simulink model "Control_System_Integrated"  (R2024a)
settings: Solver=ode23tb  StartTime=0.0  StopTime=0.1  FixedStep=1e-5  MaxStep=1e-05  RelTol=1e-3
settings Model: Creator=PME406_01  LastModifiedBy=PME406_01

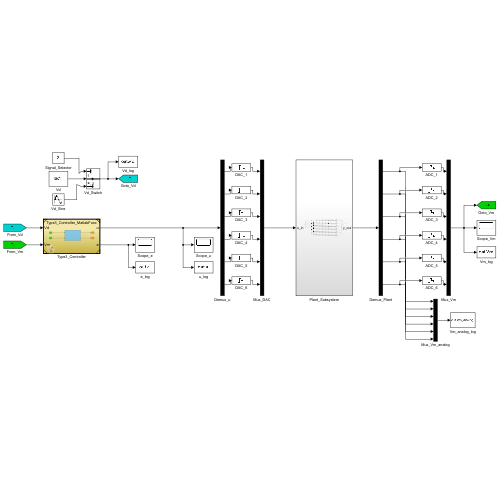
[thumbnail: Simulink's stored preview of the top-level diagram]
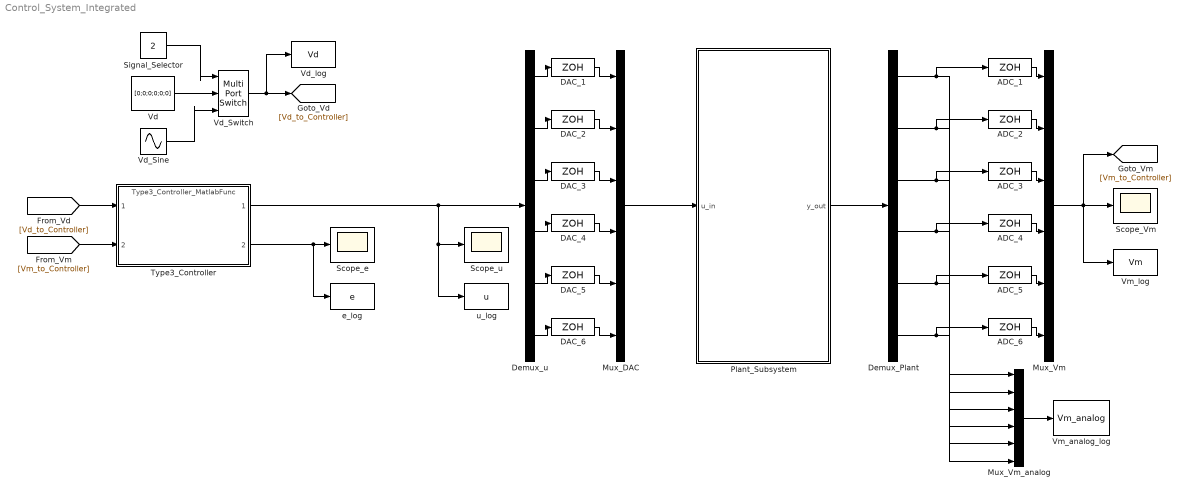
== system Control_System_Integrated ==
  ADC_{1..6} (6 alike) : ZeroOrderHold  SampleTime=1e-05
  DAC_{1..6} (6 alike) : ZeroOrderHold  SampleTime=1e-05
  Demux_Plant : Demux  Outputs=6
  Demux_u : Demux  Outputs=6
  Mux_DAC : Mux  Inputs=6
  Mux_Vm : Mux  Inputs=6
  Mux_Vm_analog : Mux  Inputs=6
  Plant_Subsystem : Subsystem
  Scope_Vm : Scope
  Scope_e : Scope
  Scope_u : Scope
  Signal_Selector : Constant  Value=2
  Type3_Controller : ModelReference  ModelNameDialog=Type3_Controller_MatlabFunc  SimulationMode=Normal  ModelReferenceVersion=1.12
  Vd : Constant  Value=[0;0;0;0;0;0]  SampleTime=1e-05
  Vd_Sine : Sin  Amplitude=[0;0;0;0;0.5;0]  Bias=[0; 0; 0; 0; 0; 0]  Frequency=3141.5927  Phase=[0;0;0;0;0;0]  SampleTime=1e-5
  Vd_Switch : MultiPortSwitch  Inputs=2  SaturateOnIntegerOverflow=off  InputSameDT=off
  Vd_log : ToWorkspace  VariableName=Vd  SampleTime=-1
      settings: Save2DSignal=2-D array (concatenate along first dimension)
  Vm_analog_log : ToWorkspace  VariableName=Vm_analog  SampleTime=-1
      settings: Save2DSignal=2-D array (concatenate along first dimension)
  Vm_log : ToWorkspace  VariableName=Vm  SampleTime=-1
      settings: Save2DSignal=2-D array (concatenate along first dimension)
  e_log : ToWorkspace  VariableName=e  SampleTime=-1
      settings: Save2DSignal=2-D array (concatenate along first dimension)
  u_log : ToWorkspace  VariableName=u  SampleTime=-1
      settings: Save2DSignal=2-D array (concatenate along first dimension)
  wires:
  Type3_Controller/1 -> u_log/1, Scope_u/1, Demux_u/1
  Demux_u/1 -> DAC_1/1
  Demux_u/2 -> DAC_2/1
  Demux_u/3 -> DAC_3/1
  Demux_u/4 -> DAC_4/1
  Demux_u/5 -> DAC_5/1
  Demux_u/6 -> DAC_6/1
  DAC_1/1 -> Mux_DAC/1
  DAC_2/1 -> Mux_DAC/2
  DAC_3/1 -> Mux_DAC/3
  DAC_4/1 -> Mux_DAC/4
  DAC_5/1 -> Mux_DAC/5
  DAC_6/1 -> Mux_DAC/6
  Plant_Subsystem/1(y_out) -> Demux_Plant/1
  Demux_Plant/1 -> ADC_1/1, Mux_Vm_analog/1
  Demux_Plant/2 -> ADC_2/1, Mux_Vm_analog/2
  Demux_Plant/3 -> ADC_3/1, Mux_Vm_analog/3
  Demux_Plant/4 -> ADC_4/1, Mux_Vm_analog/4
  Demux_Plant/5 -> ADC_5/1, Mux_Vm_analog/5
  Demux_Plant/6 -> ADC_6/1, Mux_Vm_analog/6
  ADC_1/1 -> Mux_Vm/1
  ADC_2/1 -> Mux_Vm/2
  ADC_3/1 -> Mux_Vm/3
  ADC_4/1 -> Mux_Vm/4
  ADC_5/1 -> Mux_Vm/5
  ADC_6/1 -> Mux_Vm/6
  Mux_Vm/1 -> Vm_log/1, Scope_Vm/1, [Vm_to_Controller]
  Mux_Vm_analog/1 -> Vm_analog_log/1
  Type3_Controller/2 -> e_log/1, Scope_e/1
  [Vm_to_Controller] -> Type3_Controller/2
  [Vd_to_Controller] -> Type3_Controller/1
  Vd/1 -> Vd_Switch/2
  Vd_Sine/1 -> Vd_Switch/3
  Signal_Selector/1 -> Vd_Switch/1
  Vd_Switch/1 -> Vd_log/1, [Vd_to_Controller]
  Mux_DAC/1 -> Plant_Subsystem/1(u_in)

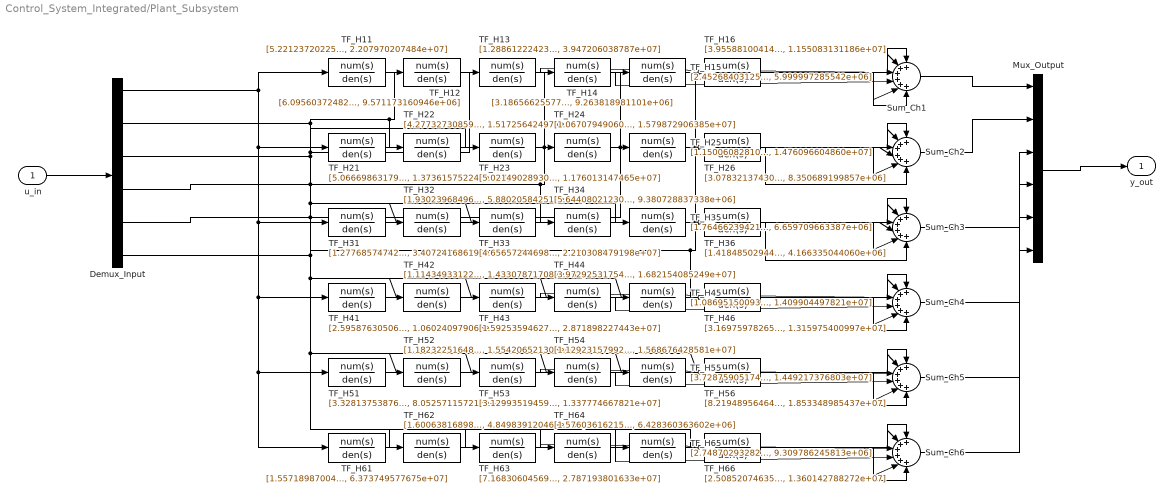
== system Control_System_Integrated/Plant_Subsystem ==
  u_in : Inport
  Demux_Input : Demux  Outputs=6
  Mux_Output : Mux  Inputs=6
  Sum_Ch{1..6} (6 alike) : Sum  Inputs=++++++
  TF_H11 : TransferFcn  Numerator=[5.221237202258e+06]  Denominator=[1, 1.125476429798e+04, 2.207970207484e+07]
  TF_H12 : TransferFcn  Numerator=[6.095603724823e+04]  Denominator=[1, 1.615096196557e+03, 9.571173160946e+06]
  TF_H13 : TransferFcn  Numerator=[1.288612224236e+06]  Denominator=[1, 1.231137597589e+04, 3.947206038787e+07]
  TF_H14 : TransferFcn  Numerator=[3.186566255776e+05]  Denominator=[1, 7.765927137710e+03, 9.263818981101e+06]
  TF_H15 : TransferFcn  Numerator=[2.452684031253e+05]  Denominator=[1, 5.746401647961e+03, 5.999997285542e+06]
  TF_H16 : TransferFcn  Numerator=[3.955881004140e+05]  Denominator=[1, 3.580306515557e+03, 1.155083131186e+07]
  TF_H21 : TransferFcn  Numerator=[5.066698631790e+04]  Denominator=[1, 1.108261849372e+03, 1.373615752245e+07]
  TF_H22 : TransferFcn  Numerator=[4.277327308593e+06]  Denominator=[1, 1.003268373777e+04, 1.517256424974e+07]
  TF_H23 : TransferFcn  Numerator=[5.021490289304e+05]  Denominator=[1, 8.810895080316e+03, 1.176013147465e+07]
  TF_H24 : TransferFcn  Numerator=[1.067079490600e+06]  Denominator=[1, 1.135112820448e+04, 1.579872906385e+07]
  TF_H25 : TransferFcn  Numerator=[1.150060828107e+06]  Denominator=[1, 1.065992916636e+04, 1.476096604860e+07]
  TF_H26 : TransferFcn  Numerator=[3.078321374306e+05]  Denominator=[1, 6.847783968129e+03, 8.350689199857e+06]
  TF_H31 : TransferFcn  Numerator=[1.277685747428e+06]  Denominator=[1, 1.368269686933e+04, 3.407241686199e+07]
  TF_H32 : TransferFcn  Numerator=[1.930239684968e+05]  Denominator=[1, 4.560870597302e+03, 5.880205842512e+06]
  TF_H33 : TransferFcn  Numerator=[4.656572446985e+06]  Denominator=[1, 9.513164457161e+03, 2.210308479198e+07]
  TF_H34 : TransferFcn  Numerator=[5.644080212304e+04]  Denominator=[1, 1.954878812118e+03, 9.380728837338e+06]
  TF_H35 : TransferFcn  Numerator=[1.764662394212e+05]  Denominator=[1, 5.122349981324e+03, 6.659709663387e+06]
  TF_H36 : TransferFcn  Numerator=[1.418485029440e+05]  Denominator=[1, 1.438504147902e+03, 4.166335044060e+06]
  TF_H41 : TransferFcn  Numerator=[2.595876305066e+05]  Denominator=[1, 7.070165651413e+03, 1.060240979066e+07]
  TF_H42 : TransferFcn  Numerator=[1.114349331223e+06]  Denominator=[1, 9.846928206402e+03, 1.433078717084e+07]
  TF_H43 : TransferFcn  Numerator=[1.592535946272e+05]  Denominator=[1, 2.790294019501e+03, 2.871898227443e+07]
  TF_H44 : TransferFcn  Numerator=[3.972925317547e+06]  Denominator=[1, 1.159715140811e+04, 1.682154085249e+07]
  TF_H45 : TransferFcn  Numerator=[1.086951500933e+06]  Denominator=[1, 1.075231371220e+04, 1.409904497821e+07]
  TF_H46 : TransferFcn  Numerator=[3.169759782656e+05]  Denominator=[1, 8.067558736035e+03, 1.315975400997e+07]
  TF_H51 : TransferFcn  Numerator=[3.328137538766e+05]  Denominator=[1, 7.227274813518e+03, 8.052571157216e+06]
  TF_H52 : TransferFcn  Numerator=[1.182322516481e+06]  Denominator=[1, 1.030784744910e+04, 1.554206521303e+07]
  TF_H53 : TransferFcn  Numerator=[3.129935194599e+05]  Denominator=[1, 7.870328655037e+03, 1.337774667821e+07]
  TF_H54 : TransferFcn  Numerator=[1.129231579925e+06]  Denominator=[1, 1.104821595243e+04, 1.568676428581e+07]
  TF_H55 : TransferFcn  Numerator=[3.728759051745e+06]  Denominator=[1, 1.050075182774e+04, 1.449217376803e+07]
  TF_H56 : TransferFcn  Numerator=[8.219489564647e+04]  Denominator=[1, 1.407969854523e+03, 1.853348985437e+07]
  TF_H61 : TransferFcn  Numerator=[1.557189870041e+06]  Denominator=[1, 2.234640585923e+04, 6.373749577675e+07]
  TF_H62 : TransferFcn  Numerator=[1.600638168987e+05]  Denominator=[1, 3.864055922471e+03, 4.849839120469e+06]
  TF_H63 : TransferFcn  Numerator=[7.168306045699e+05]  Denominator=[1, 9.251556589809e+03, 2.787193801633e+07]
  TF_H64 : TransferFcn  Numerator=[1.576036162155e+05]  Denominator=[1, 4.743270970318e+03, 6.428360363602e+06]
  TF_H65 : TransferFcn  Numerator=[2.748702932822e+04]  Denominator=[1, 4.876033357949e+02, 9.309786245813e+06]
  TF_H66 : TransferFcn  Numerator=[2.508520746356e+06]  Denominator=[1, 5.985310903650e+03, 1.360142788272e+07]
  y_out : Outport
  wires:
  u_in/1 -> Demux_Input/1
  Demux_Input/1 -> TF_H11/1, TF_H51/1, TF_H61/1, TF_H41/1, TF_H31/1, TF_H21/1
  TF_H11/1 -> Sum_Ch1/1
  Demux_Input/2 -> TF_H12/1, TF_H22/1, TF_H52/1, TF_H62/1, TF_H42/1, TF_H32/1
  TF_H12/1 -> Sum_Ch1/2
  Demux_Input/3 -> TF_H13/1, TF_H23/1, TF_H53/1, TF_H63/1, TF_H43/1, TF_H33/1
  TF_H13/1 -> Sum_Ch1/3
  Demux_Input/4 -> TF_H54/1, TF_H64/1, TF_H44/1, TF_H14/1, TF_H24/1, TF_H34/1
  TF_H14/1 -> Sum_Ch1/4
  Demux_Input/5 -> TF_H55/1, TF_H65/1, TF_H45/1, TF_H15/1, TF_H25/1, TF_H35/1
  TF_H15/1 -> Sum_Ch1/5
  Demux_Input/6 -> TF_H16/1, TF_H26/1, TF_H36/1, TF_H46/1, TF_H56/1, TF_H66/1
  TF_H16/1 -> Sum_Ch1/6
  TF_H21/1 -> Sum_Ch2/1
  TF_H22/1 -> Sum_Ch2/2
  TF_H23/1 -> Sum_Ch2/3
  TF_H24/1 -> Sum_Ch2/4
  TF_H25/1 -> Sum_Ch2/5
  TF_H26/1 -> Sum_Ch2/6
  TF_H31/1 -> Sum_Ch3/1
  TF_H32/1 -> Sum_Ch3/2
  TF_H33/1 -> Sum_Ch3/3
  TF_H34/1 -> Sum_Ch3/4
  TF_H35/1 -> Sum_Ch3/5
  TF_H36/1 -> Sum_Ch3/6
  TF_H41/1 -> Sum_Ch4/1
  TF_H42/1 -> Sum_Ch4/2
  TF_H43/1 -> Sum_Ch4/3
  TF_H44/1 -> Sum_Ch4/4
  TF_H45/1 -> Sum_Ch4/5
  TF_H46/1 -> Sum_Ch4/6
  TF_H51/1 -> Sum_Ch5/1
  TF_H52/1 -> Sum_Ch5/2
  TF_H53/1 -> Sum_Ch5/3
  TF_H54/1 -> Sum_Ch5/4
  TF_H55/1 -> Sum_Ch5/5
  TF_H56/1 -> Sum_Ch5/6
  TF_H61/1 -> Sum_Ch6/1
  TF_H62/1 -> Sum_Ch6/2
  TF_H63/1 -> Sum_Ch6/3
  TF_H64/1 -> Sum_Ch6/4
  TF_H65/1 -> Sum_Ch6/5
  TF_H66/1 -> Sum_Ch6/6
  Sum_Ch1/1 -> Mux_Output/1
  Sum_Ch2/1 -> Mux_Output/2
  Sum_Ch3/1 -> Mux_Output/3
  Sum_Ch4/1 -> Mux_Output/4
  Sum_Ch5/1 -> Mux_Output/5
  Sum_Ch6/1 -> Mux_Output/6
  Mux_Output/1 -> y_out/1
